simulink model "Feeder_0"  (R2016b)
settings: Solver=ode1  StartTime=0.0  StopTime=inf  FixedStep=Ts  RelTol=1e-3
values from neighbouring files (symbols this model uses):
  r = randi(100)    [Feeder_0_Param.m]    (also in Feeder_1_Param.m)
settings Model: Creator=sixifo  LastModifiedBy=sixifo

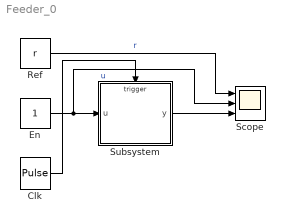
== system Feeder_0 ==
  Clk : DiscretePulseGenerator  PulseType=Time based  Period=10  PulseWidth=50
  En : Constant
  Ref : Constant  Value=r
  Scope : Scope  NumInputPorts=3
  Subsystem : Subsystem
  wires:
  En/1 -> Subsystem/1(u), Scope/2  "u"
  Ref/1 -> Scope/1  "r"
  Subsystem/1(y) -> Scope/3
  Clk/1 -> Subsystem/Trigger

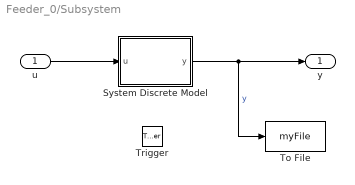
== system Feeder_0/Subsystem ==
  u : Inport
  Trigger : TriggerPort  VariantControl=Variant  PortDimensions=1
  System Discrete Model : MATLAB Function  TreatAsAtomicUnit=on
  To File : ToFile  Filename=myFile  MatrixName=yo
  y : Outport
  wires:
  u/1 -> System Discrete Model/1(u)
  System Discrete Model/1(y) -> To File/1, y/1  "y"

== matlab function Feeder_0/Subsystem/System Discrete Model ==
  data: u input; y output
function y = fcn(u)

y=u*rand*100; % Load variable stored in .mat File
